simulink model "truck_fra_oven_med_henger"  (R2019b)
settings: Solver=VariableStepAuto  StartTime=0.0  StopTime=50  MaxStep=0.01  RelTol=1e-3
settings Model: EnablePacing=on  Creator=hansae  LastModifiedBy=hansae
settings DebuggingCC: UnconnectedInputMsg=none  UnconnectedOutputMsg=none  UnconnectedLineMsg=none  SFMachineParentedDataDiag=error
settings ModelReferenceCC: EnableRefExpFcnMdlSchedulingChecks=off
settings RTWCC: Description=Generic Real-Time Target

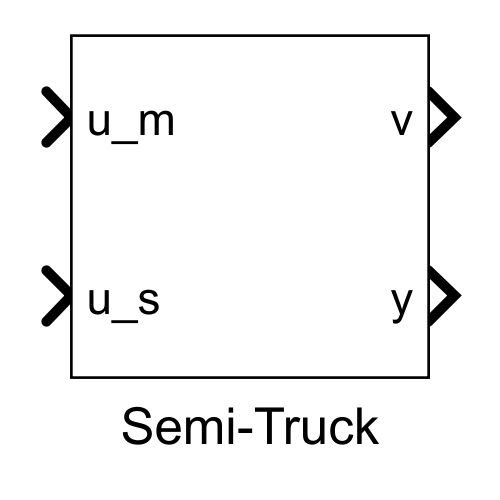
[thumbnail: Simulink's stored preview of the top-level diagram]
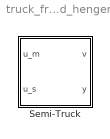
== system truck_fra_oven_med_henger ==
  Semi-Truck : Subsystem

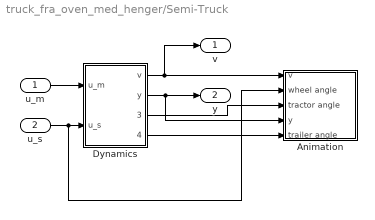
== system truck_fra_oven_med_henger/Semi-Truck ==
  u_m : Inport
  u_s : Inport  Port=2
  Animation : Subsystem
  Dynamics : Subsystem  ClipboardFcn=parameters_truck.m
  v : Outport
  y : Outport  Port=2
  wires:
  Dynamics/2(y) -> y/1, Animation/4(y)
  u_s/1 -> Animation/2(wheel angle), Dynamics/2(u_s)
  Dynamics/3(tractor angle) -> Animation/3(tractor angle)
  Dynamics/4(trailer angle) -> Animation/5(trailer angle)
  Dynamics/1(v) -> v/1, Animation/1(v)
  u_m/1 -> Dynamics/1(u_m)

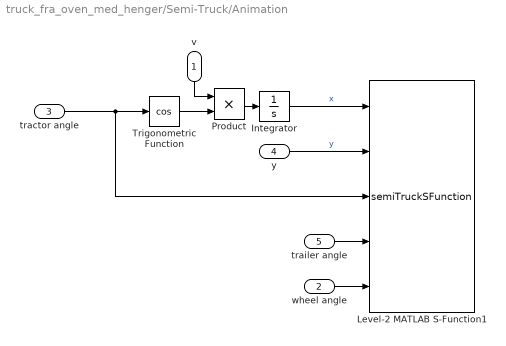
== system truck_fra_oven_med_henger/Semi-Truck/Animation ==
  v : Inport
  wheel angle : Inport  Port=2
  tractor angle : Inport  Port=3
  y : Inport  Port=4
  trailer angle : Inport  Port=5
  Integrator : Integrator
  Level-2 MATLAB S-Function1 : M-S-Function  FunctionName=semiTruckSFunction
  Product : Product
  Trigonometric Function : Trigonometry  Operator=cos
  wires:
  Product/1 -> Integrator/1
  Trigonometric Function/1 -> Product/2
  v/1 -> Product/1
  y/1 -> Level-2 MATLAB S-Function1/2  "y"
  Integrator/1 -> Level-2 MATLAB S-Function1/1  "x"
  tractor angle/1 -> Trigonometric Function/1, Level-2 MATLAB S-Function1/3
  wheel angle/1 -> Level-2 MATLAB S-Function1/5
  trailer angle/1 -> Level-2 MATLAB S-Function1/4

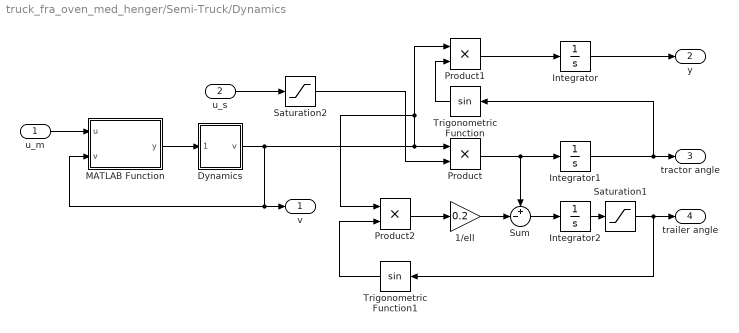
== system truck_fra_oven_med_henger/Semi-Truck/Dynamics ==
  u_m : Inport
  u_s : Inport  Port=2
  1/ell : Gain  Gain=0.2
  Dynamics : Subsystem  ClipboardFcn=parameters_truck.m
  Integrator : Integrator  InitialCondition=-2
  Integrator1 : Integrator
  Integrator2 : Integrator
  MATLAB Function : MATLAB Function  TreatAsAtomicUnit=on
  Product : Product
  Product1 : Product
  Product2 : Product
  Saturation1 : Saturate  UpperLimit=pi/2  LowerLimit=-pi/2
  Saturation2 : Saturate  UpperLimit=pi/2  LowerLimit=-pi/2
  Sum : Sum  Inputs=+-|
  Trigonometric Function : Trigonometry
  Trigonometric Function1 : Trigonometry
  v : Outport
  y : Outport  Port=2
  tractor angle : Outport  Port=3
  trailer angle : Outport  Port=4
  wires:
  Integrator/1 -> y/1
  Integrator1/1 -> tractor angle/1, Trigonometric Function/1
  Product/1 -> Integrator1/1, Sum/1
  Dynamics/1(v) -> MATLAB Function/2(v), v/1, Product2/1, Product1/1, Product/1
  Product1/1 -> Integrator/1
  Trigonometric Function/1 -> Product1/2
  Trigonometric Function1/1 -> Product2/2
  Product2/1 -> 1/ell/1
  Sum/1 -> Integrator2/1
  1/ell/1 -> Sum/2
  u_s/1 -> Saturation2/1
  Saturation2/1 -> Product/2
  Saturation1/1 -> Trigonometric Function1/1, trailer angle/1
  Integrator2/1 -> Saturation1/1
  MATLAB Function/1(y) -> Dynamics/1(u_m)
  u_m/1 -> MATLAB Function/1(u)

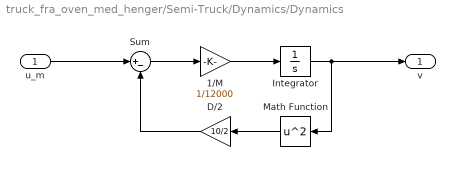
== system truck_fra_oven_med_henger/Semi-Truck/Dynamics/Dynamics ==
  u_m : Inport
  1/M : Gain  Gain=1/12000
  D/2 : Gain  Gain=10/2
  Integrator : Integrator
  Math Function : Math  Operator=square  SaturateOnIntegerOverflow=on
  Sum : Sum  Inputs=|+-
  v : Outport
  wires:
  Integrator/1 -> v/1, Math Function/1
  Sum/1 -> 1/M/1
  u_m/1 -> Sum/1
  1/M/1 -> Integrator/1
  D/2/1 -> Sum/2
  Math Function/1 -> D/2/1

== matlab function truck_fra_oven_med_henger/Semi-Truck/Dynamics/MATLAB Function ==
  data: u input; y output; v input
function y = saturation(u,v)
    Pmax = 400000;
    epsilon = 0.1;
    
    sat = Pmax/sqrt(v^2+epsilon);
    y = max(min(u,sat),-sat);
